simulink model "Q2_StaticObserverFeedback"  (R2021a)
settings: Solver=ode45  StartTime=0.0  StopTime=10.0  RelTol=1e-3
values from neighbouring files (symbols this model uses):
  A = [0 1 0 0; (m+M)*g/(M*L) 0 0 0; 0 0 0 1; (-m*g)/M 0 0 0]    [StateSpaceREP.m]
  A_observer = A - K_fast * C    [StateSpaceREP.m]
  B = [0; -1/M*L; 0; 1/M]    [StateSpaceREP.m]
  B_observer = [B K_fast]    [StateSpaceREP.m]
  C = [1 0 0 0; 0 0 1 0]    [StateSpaceREP.m]
  C_block = eye(4)    [StateSpaceREP.m]
  C_observer = eye(4)    [StateSpaceREP.m]
  D_block = zeros(4,1)    [StateSpaceREP.m]
  D_observer = zeros(4,3)    [StateSpaceREP.m]
  F = -acker(A,B,desiredEigen)    [StateSpaceREP.m]
settings Model: Creator=pbmellache2020  LastModifiedBy=pbmellache2020
settings DataIOCC: ReturnWorkspaceOutputs=off  Refine=4

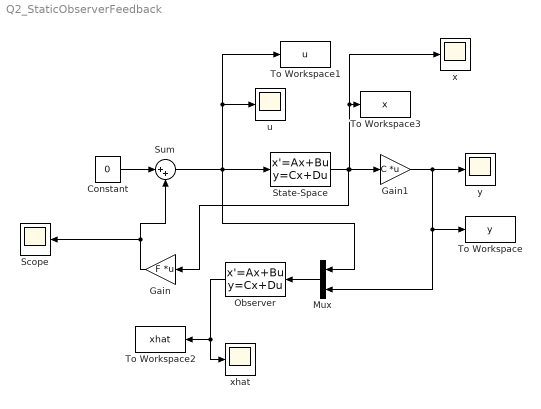
== system Q2_StaticObserverFeedback ==
  Constant : Constant  Value=0
  Gain : Gain  Gain=F  Multiplication=Matrix(K*u)
  Gain1 : Gain  Gain=C  Multiplication=Matrix(K*u)
  Mux : Mux  Inputs=2
  Observer : StateSpace  A=A_observer  B=B_observer  C=C_observer  D=D_observer  InitialCondition=[0 0 0 0]
  Scope : Scope
  State-Space : StateSpace  A=A  B=B  C=C_block  D=D_block  InitialCondition=[0.1 0 0.1 0]
  Sum : Sum  Inputs=|++
  To Workspace : ToWorkspace  VariableName=y  SampleTime=-1
  To Workspace1 : ToWorkspace  VariableName=u  SampleTime=-1
  To Workspace2 : ToWorkspace  VariableName=xhat  SampleTime=-1
  To Workspace3 : ToWorkspace  VariableName=x  SampleTime=-1
  u : Scope
  x : Scope
  xhat : Scope
  y : Scope
  wires:
  Constant/1 -> Sum/1
  Sum/1 -> Mux/1, To Workspace1/1, u/1, State-Space/1
  Mux/1 -> Observer/1
  Gain/1 -> Scope/1, Sum/2
  State-Space/1 -> Gain/1, x/1, To Workspace3/1, Gain1/1
  Gain1/1 -> Mux/2, To Workspace/1, y/1
  Observer/1 -> xhat/1, To Workspace2/1
